simulink model "test_controller"  (R2020a)
settings: Solver=ode1  StartTime=0.0  StopTime=100  FixedStep=0.01  RelTol=1e-3
InitFcn:
  | Initialization;
values from neighbouring files (symbols this model uses):
  g_I = [0 0 9.8]'    [Disturbance_rotor_payload_ini.m]    (also in Initialization.m = [0 0 g]'; parameter_verification_1drone.m = [0 0 g]')
  invJ_B1 = inv(J)    [Disturbance_rotor_payload_ini.m]    (also in Initialization.m)
  J = [2 0.3 -0.5;0.3 1 0.2;-0.5 0.2 3]*10^-2    [Disturbance_rotor_payload_ini.m]    (also in Initialization.m)
  K_0 = 5    [Initialization.m]
  k_L = 0.15    [Initialization.m]
  K_omega = 1*eye(3)    [Disturbance_rotor_payload_ini.m]    (also in Initialization.m)
  k_p = 0.10    (= 0.1)    [Initialization.m]
  K_q = 100    [Disturbance_rotor_payload_ini.m]    (also in Initialization.m)
  K_R = 1*eye(3)    [Disturbance_rotor_payload_ini.m]    (also in Initialization.m)
  k_v = 7    [Disturbance_rotor_payload_ini.m]    (also in Initialization.m = 0.24)
  kappa = 0.9    [Initialization.m]
  Kr = 0.2    [Initialization.m]    (also in parameter_verification_1drone.m)
  L = 1    [Disturbance_rotor_payload_ini.m]    (also in Initialization.m = 0.98; parameter_verification_1drone.m = 0.98)
  Lambda = 0.4    [Initialization.m]    (also in parameter_verification_1drone.m)
  Lambda_initalB01 = angle2quat(initial_Euler(3),initial_Euler(2),initial_Euler(1))    [Disturbance_rotor_payload_ini.m]    (also in Initialization.m)
  lambda_p = 0.2    [Disturbance_rotor_payload_ini.m]    (also in Initialization.m)
  lambda_q = 0.3    [Disturbance_rotor_payload_ini.m]    (also in Initialization.m)
  Lambda_T = 0.5    [Initialization.m]
  m_p = 0.5    [Disturbance_rotor_payload_ini.m]    (also in Initialization.m; parameter_verification_1drone.m)
  m_q = 1.63    [Disturbance_rotor_payload_ini.m]    (also in Initialization.m)
  n_1 = [0 1 0]'    [Disturbance_rotor_payload_ini.m]    (also in Initialization.m)
  omega_b01 = [0.1 0.3 0]'    [Disturbance_rotor_payload_ini.m]    (also in Initialization.m)
  P_1 = [5 0 -6]'    [Disturbance_rotor_payload_ini.m]    (also in Initialization.m)
  U_initial = [y_dot_initial;v_q]    [Disturbance_rotor_payload_ini.m]    (also in Initialization.m)
  W_p = [-0.4 0.8 -0.3]'    [Disturbance_rotor_payload_ini.m]    (also in Initialization.m)
  W_q = [-1 2 -0.3]'    [Disturbance_rotor_payload_ini.m]    (also in Initialization.m)
  X_initial = [0 0 0]'    [Disturbance_rotor_payload_ini.m]    (also in Initialization.m)
  y_inital = [0.02 -0.02]'    [Disturbance_rotor_payload_ini.m]    (also in Initialization.m)
libraries: sharedtransform x2, dspinverses x2, dspmtrx3 x1, sharedutil x1
(part 2 of 2)

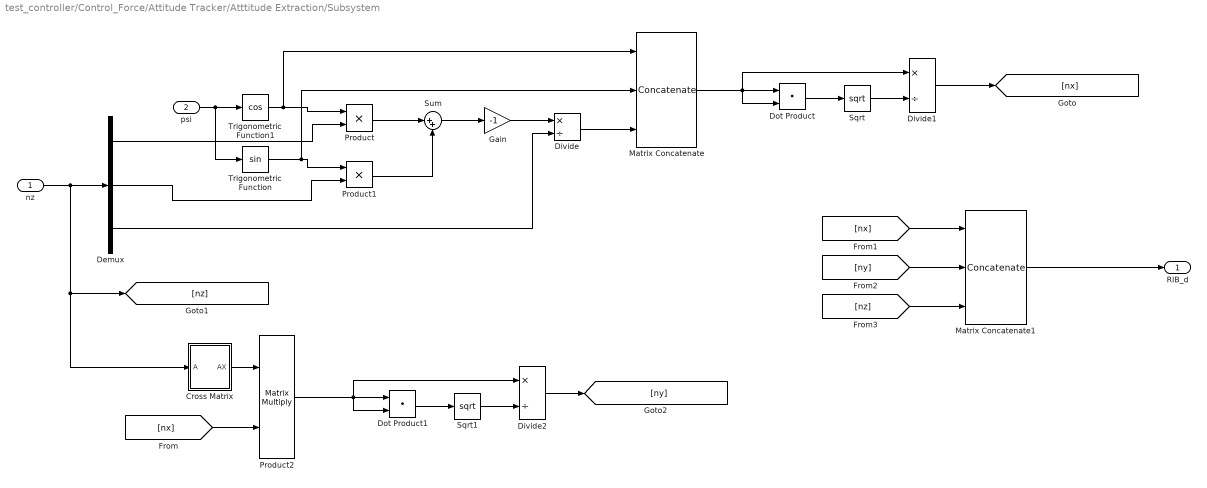
== system test_controller/Control_Force/Attitude Tracker/Atttitude Extraction/Subsystem ==
  nz : Inport
  psi : Inport  Port=2
  Cross Matrix : Subsystem
  Demux : Demux  Outputs=3
  Divide : Product  Inputs=*/
  Divide1 : Product  Inputs=*/
  Divide2 : Product  Inputs=*/
  Dot Product : DotProduct  InputSameDT=on  OutDataTypeStr=Inherit: Inherit via internal rule
  Dot Product1 : DotProduct  InputSameDT=on  OutDataTypeStr=Inherit: Inherit via internal rule
  Gain : Gain  Gain=-1
  Matrix Concatenate : Concatenate  NumInputs=3  Mode=Multidimensional array
  Matrix Concatenate1 : Concatenate  NumInputs=3  Mode=Multidimensional array  ConcatenateDimension=2
  Product : Product
  Product1 : Product
  Product2 : Product  Multiplication=Matrix(*)
  Sqrt : Sqrt  SaturateOnIntegerOverflow=on
  Sqrt1 : Sqrt  SaturateOnIntegerOverflow=on
  Sum : Sum  Inputs=|++
  Trigonometric Function : Trigonometry
  Trigonometric Function1 : Trigonometry  Operator=cos
  RIB_d : Outport  VectorParamsAs1DForOutWhenUnconnected=off
  wires:
  nz/1 -> Cross Matrix/1(A), [nz], Demux/1
  Demux/1 -> Product/2
  Demux/3 -> Divide/2
  psi/1 -> Trigonometric Function/1, Trigonometric Function1/1
  Trigonometric Function1/1 -> Matrix Concatenate/1, Product/1
  Trigonometric Function/1 -> Matrix Concatenate/2, Product1/1
  Demux/2 -> Product1/2
  Product/1 -> Sum/1
  Product1/1 -> Sum/2
  Sum/1 -> Gain/1
  Gain/1 -> Divide/1
  Divide/1 -> Matrix Concatenate/3
  Matrix Concatenate/1 -> Divide1/1, Dot Product/1, Dot Product/2
  Dot Product/1 -> Sqrt/1
  Sqrt/1 -> Divide1/2
  Divide1/1 -> [nx]
  Cross Matrix/1(AX) -> Product2/1
  [nx] -> Product2/2
  [nx] -> Matrix Concatenate1/1
  [ny] -> Matrix Concatenate1/2
  [nz] -> Matrix Concatenate1/3
  Product2/1 -> Divide2/1, Dot Product1/1, Dot Product1/2
  Dot Product1/1 -> Sqrt1/1
  Sqrt1/1 -> Divide2/2
  Divide2/1 -> [ny]
  Matrix Concatenate1/1 -> RIB_d/1

== system test_controller/Control_Force/Attitude Tracker/Atttitude Extraction/vee map ==
  skrew symmetric matrix : Inport
  Display2 : Display
  Display3 : Display
  Mux : Mux  Inputs=3
  Selector : Selector  NumberOfDimensions=2  InputPortWidth=3  IndexOptions=Index vector (dialog),Index vector (dialog)  Indices=3,2  OutputSizes=1,1
  Selector1 : Selector  NumberOfDimensions=2  InputPortWidth=3  IndexOptions=Index vector (dialog),Index vector (dialog)  Indices=1,3  OutputSizes=1,1
  Selector2 : Selector  NumberOfDimensions=2  InputPortWidth=3  IndexOptions=Index vector (dialog),Index vector (dialog)  Indices=2,1  OutputSizes=1,1
  phi : Outport  VectorParamsAs1DForOutWhenUnconnected=off
  wires:
  skrew symmetric matrix/1 -> Selector/1, Display3/1, Selector2/1, Selector1/1
  Mux/1 -> phi/1, Display2/1
  Selector/1 -> Mux/1
  Selector1/1 -> Mux/2
  Selector2/1 -> Mux/3

== system test_controller/Control_Force/Attitude Tracker/Attitude Dynamics/Quaternion Based Attitude Calculation/L_hat ==
  Lambda : Inport
  Create Diagonal Matrix1 : dspmtrx3/Create Diagonal Matrix
      settings: SourceProductBaseCode=DS
  Cross Matrix : Subsystem
  Gain : Gain  Gain=-1
  Gain1 : Gain  Gain=[1 1 1]
  Gain2 : Gain  Gain=-1
  Matrix Concatenate : Concatenate  Mode=Multidimensional array  ConcatenateDimension=2
  Selector : Selector  InputPortWidth=4  IndexOptions=Index vector (dialog)  Indices=[2 3 4]  OutputSizes=1
  Selector1 : Selector  InputPortWidth=4  IndexOptions=Index vector (dialog)  Indices=[1]  OutputSizes=1
  Sum : Sum  Inputs=|++
  L_hat : Outport  VectorParamsAs1DForOutWhenUnconnected=off
  wires:
  Lambda/1 -> Selector/1, Selector1/1
  Gain/1 -> Matrix Concatenate/1
  Matrix Concatenate/1 -> L_hat/1
  Cross Matrix/1(AX) -> Gain2/1  "LambdaX"
  Sum/1 -> Matrix Concatenate/2
  Selector1/1 -> Gain1/1
  Gain1/1 -> Create Diagonal Matrix1/1
  Selector/1 -> Cross Matrix/1(A), Gain/1
  Create Diagonal Matrix1/1 -> Sum/2
  Gain2/1 -> Sum/1

== system test_controller/Control_Force/Attitude Tracker/Atttitude Extraction/Subsystem/Cross Matrix ==
  A : Inport
  Constant1 : Constant  Value=0  VectorParams1D=off
  Constant2 : Constant  Value=0  VectorParams1D=off
  Constant3 : Constant  Value=0  VectorParams1D=off
  Demux2 : Demux  Outputs=3
  Gain : Gain  Gain=-1
  Gain1 : Gain  Gain=-1
  Gain2 : Gain  Gain=-1
  Matrix Concatenate : Concatenate  NumInputs=3  Mode=Multidimensional array  ConcatenateDimension=2
  Matrix Concatenate1 : Concatenate  NumInputs=3  Mode=Multidimensional array
  Matrix Concatenate2 : Concatenate  NumInputs=3  Mode=Multidimensional array
  Matrix Concatenate3 : Concatenate  NumInputs=3  Mode=Multidimensional array
  AX : Outport  VectorParamsAs1DForOutWhenUnconnected=off
  wires:
  A/1 -> Demux2/1
  Demux2/1 -> Gain1/1, Matrix Concatenate2/3  "r1"
  Demux2/2 -> Gain2/1, Matrix Concatenate3/1  "r2"
  Matrix Concatenate/1 -> AX/1
  Demux2/3 -> Gain/1, Matrix Concatenate1/2  "r3"
  Matrix Concatenate1/1 -> Matrix Concatenate/1
  Matrix Concatenate2/1 -> Matrix Concatenate/2
  Constant2/1 -> Matrix Concatenate2/2
  Gain/1 -> Matrix Concatenate2/1
  Matrix Concatenate3/1 -> Matrix Concatenate/3
  Gain1/1 -> Matrix Concatenate3/2
  Constant3/1 -> Matrix Concatenate3/3
  Constant1/1 -> Matrix Concatenate1/1
  Gain2/1 -> Matrix Concatenate1/3

== system test_controller/Control_Force/Attitude Tracker/Attitude Dynamics/Quaternion Based Attitude Calculation/L_hat/Cross Matrix ==
  A : Inport
  Constant1 : Constant  Value=0
  Constant2 : Constant  Value=0
  Constant3 : Constant  Value=0
  Demux2 : Demux  Outputs=3
  Gain : Gain  Gain=-1
  Gain1 : Gain  Gain=-1
  Gain2 : Gain  Gain=-1
  Matrix Concatenate : Concatenate  NumInputs=3  Mode=Multidimensional array  ConcatenateDimension=2
  Mux : Mux  Inputs=3
  Mux1 : Mux  Inputs=3
  Mux2 : Mux  Inputs=3
  AX : Outport  VectorParamsAs1DForOutWhenUnconnected=off
  wires:
  A/1 -> Demux2/1
  Demux2/1 -> Mux1/3, Gain1/1  "r1"
  Demux2/2 -> Mux2/1, Gain2/1  "r2"
  Matrix Concatenate/1 -> AX/1
  Demux2/3 -> Gain/1, Mux/2  "r3"
  Mux/1 -> Matrix Concatenate/1
  Mux1/1 -> Matrix Concatenate/2
  Constant2/1 -> Mux1/2
  Gain/1 -> Mux1/1
  Mux2/1 -> Matrix Concatenate/3
  Gain1/1 -> Mux2/2
  Constant3/1 -> Mux2/3
  Constant1/1 -> Mux/1
  Gain2/1 -> Mux/3
